simulink model "maze_line_path_simulation_new"  (R2020a)
settings: Solver=FixedStepAuto  StartTime=0.0  StopTime=48.4  FixedStep=0.01  RelTol=1e-3  EnableMultiTasking=on
PreLoadFcn:
  | robotParameters_maze;
values from neighbouring files (symbols this model uses):
  axleLength = 0.0672    [robotParameters_maze.m]
  J = 0.0001    [robotParameters_maze.m]
  Kb = 0.190    (= 0.19)    [robotParameters_maze.m]
  Kf = 0.000025    (= 2.5e-05)    [robotParameters_maze.m]
  Km = 0.084    [robotParameters_maze.m]
  L = 0.5    [robotParameters_maze.m]
  mapForSim =     [maze_map.mat]    (also in oval_line_map.mat)
  motorIP = [-12 -11.9 -11.8 -11.7 -11.6 -11.5 -11.4 -11.3 -11.2 -11.1 -11 -10.9 ... (241 elements, 1x241)]    [motorLUT.mat]
  motorSP = [-62.7865560716 -62.2538153955 -61.7309054619 -61.2077148683 -60.684548166 -60.1613790322 -59.6382101464 -59.1150412352 -58.5918723266 -58.0687034178 -57.545534509 -57.0223656001 ... (241 elements, 1x241)]    [motorLUT.mat]
  R = 16    [robotParameters_maze.m]
  wheelR = 0.017    [robotParameters_maze.m]
undefined symbols (not defined in the file or in its folder): DiscIntNeverNeededParam, lineLength
libraries: simulink x6, mobileRoboticsTrainingLib x2, sldrtlib x1
(part 2 of 2)

== stateflow chart maze_line_path_simulation_new/STATEFLOW LOGIC ==
  state DRY_RUN
    state CHECK_T_intersection1
      entry:
      path(i+1)=1;
      i = i + 1;
    state STOP
      entry:
      v=0;
      w=0;
      maze=path;
      solve_maze=1;
    state CHECK_cross_intersection
      entry:
      path(i+1)=1;
      i = i + 1;
    state GO_LEFT
      entry:
      v=0;
      w=ang_vel;
    state Check_intersection_or_MazeEnd
      entry:
      v=velocity;
    state Left_T_intersection
      entry:
      path(i+1)=1;
      i=i+1;
    state Left_only
    state uturn
      entry:
      v=velocity/8;
    state Check_left_only_or_left_T
      entry:
      v=velocity;
    state U_TURN
      entry:
      v=0;
      w=ang_vel;
    state Follow_Line
      entry:
      v=velocity;
      w=0;
      during:
      w=average(LF,LM,LC,RC,RM,RF);
      exit:
      w=0;
      state y = average(LF,LM,LC,RC,RM,RF) [function]
    state Check_rightonly_rightT
      entry:
      v=velocity;
    state GO_RIGHT
      entry:
      v=0;
      w=-ang_vel;
    DRY_RUN.Check_intersection_or_MazeEnd -> DRY_RUN.CHECK_T_intersection1 [order 3] : after(delay_dist,sec)[ line_pos==5]
    DRY_RUN.CHECK_T_intersection1 -> DRY_RUN.GO_LEFT
    DRY_RUN.Check_intersection_or_MazeEnd -> DRY_RUN.CHECK_cross_intersection [order 1] : after(delay_dist,sec)
        | [ line_pos==1]
    DRY_RUN.Check_intersection_or_MazeEnd -> DRY_RUN.STOP [order 2] : after(0.4,sec)
        | [line_pos==4]
    DRY_RUN.CHECK_cross_intersection -> DRY_RUN.GO_LEFT
    DRY_RUN.GO_LEFT -> DRY_RUN.Follow_Line : after(delay_turn,sec)
        |  [line_pos==1]
    DRY_RUN.Left_T_intersection -> DRY_RUN.GO_LEFT
    DRY_RUN.Left_only -> DRY_RUN.GO_LEFT
    DRY_RUN.Follow_Line -> DRY_RUN.Check_intersection_or_MazeEnd [order 3] : [line_pos==4]
    DRY_RUN.Follow_Line -> uturn [order 4] : [duration(line_pos==5) > 0.15]
    DRY_RUN.Check_left_only_or_left_T -> DRY_RUN.Left_only [order 2] : after(delay_dist,sec)
        | [line_pos==5&& RC==0 && LC==0]
    DRY_RUN.Check_left_only_or_left_T -> DRY_RUN.Left_T_intersection [order 1] : after(delay_dist,sec)
        | [line_pos==1||RC==1||LC==1]
    uturn -> DRY_RUN.Follow_Line [order 1] : [line_pos==1]
    uturn -> DRY_RUN.U_TURN [order 2] : after(0.2,sec) [line_pos==5]
        | {v=velocity/8}
    (default) -> DRY_RUN.Follow_Line : {i=0;}
    DRY_RUN.Follow_Line -> DRY_RUN.Check_left_only_or_left_T [order 1] : [line_pos==2]
    DRY_RUN.U_TURN -> DRY_RUN.Follow_Line : after(1,sec)[line_pos==1]
        | {v=0;path(i+1)=4;i = i + 1;}
    DRY_RUN.Follow_Line -> DRY_RUN.Check_rightonly_rightT [order 2] : [line_pos==3]
    DRY_RUN.GO_RIGHT -> DRY_RUN.Follow_Line : after(delay_turn,sec) [line_pos==1]
    DRY_RUN.Check_rightonly_rightT -> DRY_RUN.Follow_Line [order 2] : after(delay_dist,sec) [line_pos==1||RC==1||LC==1]
        | {path(i+1)=3;i = i + 1;}
    DRY_RUN.Check_rightonly_rightT -> DRY_RUN.GO_RIGHT [order 1] : after(delay_dist,sec)
        | [line_pos==5 && RC==0 && LC==0]
  state SHORTEST_RUN
    state GO_RIGHT
      entry:
      v=0;
      w=-ang_vel;
    state CHECK_T_intersection1
      entry:
      j=j+1;
    state GO_LEFT
      entry:
      v=0;
      w=ang_vel;
    state CHECK_cross_intersection
      entry:
      j=j+1;
    state STOP
      entry:
      v=0;
      w=0;
    state Left_only
    state Check_intersection_or_MazeEnd
      entry:
      v=velocity;
    state Follow_Line
      entry:
      v=velocity;
      w=0;
      during:
      w=fastaverage(LF,LM,LC,RC,RM,RF);
      exit:
      w=0;
      state y = fastaverage(LF,LM,LC,RC,RM,RF) [function]
    state Left_T_intersection
      entry:
      j = j + 1;
    state Right_T_intersection
      entry:
      j=j+1;
    state Right_only
    state Check_rightonly_rightT
      entry:
      v=velocity;
    state Check_left_only_or_left_T
      entry:
      v=velocity;
    (junction 199) -> SHORTEST_RUN.GO_LEFT [order 2] : [solvedpath(j)==1]
    (junction 199) -> SHORTEST_RUN.GO_RIGHT [order 1] : [solvedpath(j)==2]
    SHORTEST_RUN.CHECK_T_intersection1 -> (junction 199)
    Right_only -> SHORTEST_RUN.GO_RIGHT
    (junction 196) -> SHORTEST_RUN.GO_RIGHT [order 3] : [solvedpath(j)==2]
    SHORTEST_RUN.GO_RIGHT -> SHORTEST_RUN.Follow_Line : after(delay_turn,sec)
        | [line_pos==1]
    SHORTEST_RUN.Check_intersection_or_MazeEnd -> SHORTEST_RUN.CHECK_T_intersection1 [order 2] : after(delay_dist,sec)
        | [ line_pos==5]
    (junction 209) -> SHORTEST_RUN.GO_RIGHT [order 1] : [solvedpath(j)==2]
    (junction 194) -> SHORTEST_RUN.GO_LEFT [order 2] : [solvedpath(j)==1]
    (junction 196) -> SHORTEST_RUN.GO_LEFT [order 1] : [solvedpath(j)==1]
    SHORTEST_RUN.CHECK_cross_intersection -> (junction 196)
    (junction 196) -> SHORTEST_RUN.Follow_Line [order 2] : [solvedpath(j)==3]
    SHORTEST_RUN.Left_only -> SHORTEST_RUN.GO_LEFT
    SHORTEST_RUN.GO_LEFT -> SHORTEST_RUN.Follow_Line : after(delay_turn,sec)
        | [line_pos==1]
    SHORTEST_RUN.Check_intersection_or_MazeEnd -> SHORTEST_RUN.CHECK_cross_intersection [order 1] : after(delay_dist,sec)
        | [ line_pos==1||RC==1||LC==1]
    SHORTEST_RUN.Check_intersection_or_MazeEnd -> SHORTEST_RUN.STOP [order 3] : after(0.5,sec)
        | [line_pos==4]{w=0}
    SHORTEST_RUN.Check_left_only_or_left_T -> SHORTEST_RUN.Left_only [order 1] : after(delay_dist,sec)
        | [line_pos==5&& RC==0 && LC==0]
    (default) -> SHORTEST_RUN.Follow_Line : {j=0}
    SHORTEST_RUN.Follow_Line -> SHORTEST_RUN.Check_intersection_or_MazeEnd [order 2] : [line_pos==4]
    (junction 209) -> SHORTEST_RUN.Follow_Line [order 2] : [solvedpath(j)==3]
    (junction 194) -> SHORTEST_RUN.Follow_Line [order 1] : [solvedpath(j)==3]
    Right_T_intersection -> (junction 209)
    SHORTEST_RUN.Left_T_intersection -> (junction 194)
    SHORTEST_RUN.Follow_Line -> SHORTEST_RUN.Check_left_only_or_left_T [order 1] : [line_pos==2]
    SHORTEST_RUN.Follow_Line -> SHORTEST_RUN.Check_rightonly_rightT [order 3] : [line_pos==3]
    SHORTEST_RUN.Check_left_only_or_left_T -> SHORTEST_RUN.Left_T_intersection [order 2] : after(delay_dist,sec)
        | [line_pos==1||RC==1||LC==1]
    SHORTEST_RUN.Check_rightonly_rightT -> Right_T_intersection [order 2] : after(delay_dist,sec)
        | [line_pos==1||RC==1||LC==1]
    SHORTEST_RUN.Check_rightonly_rightT -> Right_only [order 1] : after(delay_dist,sec)
        | [line_pos==5&& RC==0 && LC==0]
  state GO_LEFT [commented out]
    entry:
    v=0;
    w=1;
  state GO_RIGHT [commented out]
    entry:
    v=0;
    w=-1;
  state Left_T_intersection [commented out]
    entry:
    path(i+1)=1;
    i=i+1;
  state Left_only [commented out]
  state Follow_Line32 [commented out]
    entry:
    v=velocity;
    w=0;
    during:
    w=average(LF,LM,LC,RC,RM,RF);
    exit:
    w=0;
    state y = average(LF,LM,LC,RC,RM,RF) [function] [commented out]
  state Follow_Line2 [commented out]
    entry:
    v=velocity;
    w=0;
    during:
    w=average(LF,LM,LC,RC,RM,RF);
    exit:
    w=0;
    state y = average(LF,LM,LC,RC,RM,RF) [function] [commented out]
  state Check_rightonly_rightT [commented out]
    entry:
    v=velocity;
  state Check_left_only_or_left_T [commented out]
    entry:
    v=velocity;
  state CHECK_cross_intersection [commented out]
    entry:
    path(i+1)=1;
    i = i + 1;
  state Check_intersection_or_MazeEnd [commented out]
    entry:
    v=velocity;
  state STOP [commented out]
    entry:
    v=0;
    w=0;
    maze=path;
    solve_maze=1;
  state GO_LEFT12 [commented out]
    entry:
    v=0;
    w=1;
  state Follow_Line14 [commented out]
    entry:
    v=velocity;
    w=0;
    during:
    w=average(LF,LM,LC,RC,RM,RF);
    exit:
    w=0;
    state y = average(LF,LM,LC,RC,RM,RF) [function] [commented out]
  state Follow_Line123 [commented out]
    entry:
    v=velocity;
    w=0;
    during:
    w=average(LF,LM,LC,RC,RM,RF);
    exit:
    w=0;
    state y = average(LF,LM,LC,RC,RM,RF) [function] [commented out]
  state U_TURN [commented out]
    entry:
    v=0;
    w=1;
  state CHECK_T_intersection [commented out]
    entry:
    path(i+1)=1;
    i = i + 1;
  (default) -> DRY_RUN
  DRY_RUN -> SHORTEST_RUN : [mode==1]
  Left_T_intersection -> GO_LEFT [commented out]
  GO_LEFT -> Follow_Line2 [commented out] : after(delay_turn,sec) [line_pos==1]
  Left_only -> GO_LEFT [commented out]
  GO_RIGHT -> Follow_Line32 [commented out] : after(delay_turn,sec) [line_pos==1]
  (default) -> Follow_Line32 [commented out] : {i=0;}
  Check_rightonly_rightT -> GO_RIGHT [commented out] : after(delay_dist,sec)
      | [line_pos==5 && RC==0 && LC==0]
  Check_left_only_or_left_T -> Left_only [commented out] : after(delay_dist,sec)
      | [line_pos==5&& RC==0 && LC==0]
  (default) -> Follow_Line2 [commented out] : {i=0;}
  Check_left_only_or_left_T -> Left_T_intersection [commented out] : after(delay_dist,sec)
      | [line_pos==1||RC==1||LC==1]
  Follow_Line32 -> Check_rightonly_rightT [commented out] : [line_pos==3]
  Follow_Line2 -> Check_left_only_or_left_T [commented out] : [line_pos==2]
  Check_rightonly_rightT -> Follow_Line32 [commented out] : after(delay_dist,sec) [line_pos==1||RC==1||LC==1]
      | {path(i+1)=3;i = i + 1;}
  SHORTEST_RUN -> DRY_RUN : [mode==0]
  Check_intersection_or_MazeEnd -> STOP [commented out] : after(0.4,sec)[line_pos==4] {w=0}
  Check_intersection_or_MazeEnd -> CHECK_cross_intersection [commented out] : after(delay_dist,sec)[ line_pos==1||RC==1||LC==1]
  CHECK_cross_intersection -> GO_LEFT12 [commented out]
  Check_intersection_or_MazeEnd -> CHECK_T_intersection [commented out] : after(delay_dist,sec)[ line_pos==5]
  Follow_Line14 -> Check_intersection_or_MazeEnd [commented out] : [line_pos==4]
  (default) -> Follow_Line14 [commented out] : {i=0;}
  (default) -> Follow_Line123 [commented out] : {i=0;}
  CHECK_T_intersection -> GO_LEFT12 [commented out]
  U_TURN -> Follow_Line123 [commented out] : after(delay_turn,sec)[line_pos==1]
      | {v=0;path(i+1)=4;i = i + 1;}
  Follow_Line123 -> U_TURN [commented out] : [duration(line_pos==5) > 1]
  data: LF function_input double size=1; y function_output; LM function_input double size=1; LC function_input double size=1; RC function_input double size=1; RM function_input double size=1; RF function_input double size=1; LF function_input double size=1; y function_output; LM function_input double size=1; LC function_input double size=1; RC function_input double size=1; RM function_input double size=1; RF function_input double size=1; LF function_input double size=1; y function_output double size=1; LM function_input double size=1; LC function_input double size=1; RC function_input double size=1; RM function_input double size=1; RF function_input double size=1; LF function_input double size=1; y function_output double size=1; LM function_input double size=1; LC function_input double size=1; RC function_input double size=1; RM function_input double size=1; RF function_input double size=1; LF function_input double size=1; y function_output double size=1; LM function_input double size=1; LC function_input double size=1; RC function_input double size=1; RM function_input double size=1; RF function_input double size=1; LF function_input double size=1; y function_output double size=1; LM function_input double size=1; LC function_input double size=1; RC function_input double size=1; RM function_input double size=1; RF function_input double size=1; LF input; LM input; LC input; RC input; RM input; RF input; velocity input; v output; w output; line_pos input; delay_dist input; delay_turn input; i local double =0; solve_maze local double =0; mode input; solvedpath input single size=[1 20]; j local double =0; path output single size=[1 20]; maze output single size=[1 20]; ang_vel input

== matlab function maze_line_path_simulation_new/Robot Simulator/MATLAB Function ==
  data: x input; y input; theta input; lineLength input
function plotRobot(x,y,theta,lineLength)
% Get plot details
coder.extrinsic('evalin','plot')
ph1 = evalin('base','PlotHandle1');
ph2 = evalin('base','PlotHandle2');

% Find length orientation line
xp = [x x+lineLength*cos(theta)];
yp = [y y+lineLength*sin(theta)];

% Plot robot
set(ph1,'xdata',xp,'ydata',yp);
set(ph2,'xdata',x,'ydata',y);
drawnow('limitrate')
